simulink model "mapp_4_fir_4_str"  (R2018b)
settings: Solver=ode45  StartTime=0.0  StopTime=200  RelTol=1e-3  EnableMultiTasking=on
undefined symbols (not defined in the file or in its folder): CMD_ci_Re_0, CMD_ci_Re_21, CMD_ci_str_0, CMD_ci_str_1, CMD_ci_str_10, CMD_ci_str_11, CMD_ci_str_12, CMD_ci_str_13, CMD_ci_str_14, CMD_ci_str_15, CMD_ci_str_16, CMD_ci_str_17, CMD_ci_str_18, CMD_ci_str_19, CMD_ci_str_2, CMD_ci_str_20, CMD_ci_str_21, CMD_ci_str_3, CMD_ci_str_4, CMD_ci_str_5, CMD_ci_str_6, CMD_ci_str_7, CMD_ci_str_8, CMD_ci_str_9, CMD_decr_0, CMD_deka_down, CMD_deka_up, CMD_fb, CMD_FB_mult, CMD_Firprg_0, CMD_Firprg_1, CMD_gain, CMD_ind_mult, CMD_ind_mult_1, CMD_ind_mult_2, CMD_ind_mult_3, CMD_ind_mult_4, CMD_ind_stuk, CMD_ind_vol, CMD_ind_vol_1, CMD_ind_vol_2, CMD_ind_vol_3, CMD_ind_vol_4, CMD_init_dac, CMD_init_sw, CMD_molot_string, CMD_nl, CMD_nl_sl, CMD_omega_0, CMD_out_vol, CMD_param_0, CMD_param_5, CMD_pedal, CMD_reset, CMD_rst, CMD_shape_0, CMD_step_down, CMD_step_up, CMD_str_svertk, ind_mult_0 ... (+10)
libraries: xbsIndex_r4 x3300
(part 12 of 16)

== system mapp_4_fir_4_str/Mid_Graph2/Exp/exp-mashinka/gauss0 ==
  sync : Inport
  addr : Inport  Port=2
  Force_vol : Inport  Port=3
  m_data : Inport  Port=4
  m_addr : Inport  Port=5
  m_en : Inport  Port=6
  Addr_ind_vol : Inport  Port=7
  AddSub : xbsIndex_r4/AddSub  mode=Subtraction  use_carryin=off  use_carryout=off  en=off  latency=2  precision=Full  arith_type=Unsigned  n_bits=16  bin_pt=14  quantization=Truncate  overflow=Wrap  use_behavioral_HDL=off  hw_selection=Fabric  pipelined=off  dbl_ovrd=off  block_type=addsub
  Constant1 : xbsIndex_r4/Constant  const=0  gui_display_data_type=Floating-point  arith_type=Floating-point  n_bits=30  bin_pt=0  preci_type=Single  exp_width=8  frac_width=24  explicit_period=on  period=1  equ=P=C  opselect=C  inp2=PCIN>>17  opr=+  inp1=P  carry=CIN  dbl_ovrd=off  block_type=constant
  Constant2 : xbsIndex_r4/Constant  const=30  gui_display_data_type=Floating-point  arith_type=Floating-point  n_bits=16  bin_pt=14  preci_type=Single  exp_width=8  frac_width=24  explicit_period=on  period=1  equ=P=C  opselect=C  inp2=PCIN>>17  opr=+  inp1=P  carry=CIN  dbl_ovrd=off  block_type=constant
  Convert : xbsIndex_r4/Convert  gui_display_data_type=Floating-point  arith_type=Floating-point  n_bits=16  bin_pt=14  float_type=Single  exp_bits=8  fraction_bits=24  quantization=Truncate  overflow=Wrap  en=off  latency=3  pipeline=off  dbl_ovrd=off  block_type=convert
  Convert2 : xbsIndex_r4/Convert  gui_display_data_type=Floating-point  arith_type=Floating-point  n_bits=16  bin_pt=14  float_type=Single  exp_bits=8  fraction_bits=24  quantization=Truncate  overflow=Wrap  en=off  latency=3  pipeline=off  dbl_ovrd=off  block_type=convert
  Convert4 : xbsIndex_r4/Convert  gui_display_data_type=Floating-point  arith_type=Floating-point  n_bits=16  bin_pt=14  float_type=Single  exp_bits=8  fraction_bits=24  quantization=Truncate  overflow=Wrap  en=off  latency=3  pipeline=off  dbl_ovrd=off  block_type=convert
  Delay1 : xbsIndex_r4/Delay  rst=off  infoeditControl=Selection of Reset will increase slice count due to use of real FFs and instead of SRLs  en=off  latency=9  reg_retiming=off  dbl_ovrd=off  block_type=delay
  Delay{2..10,14,18} (11 alike) : xbsIndex_r4/Delay  rst=off  infoeditControl=Selection of Reset will increase slice count due to use of real FFs and instead of SRLs  en=off  latency=1  reg_retiming=off  dbl_ovrd=off  block_type=delay
  Delay11 : xbsIndex_r4/Delay  rst=off  infoeditControl=Selection of Reset will increase slice count due to use of real FFs and instead of SRLs  en=off  latency=14  reg_retiming=off  dbl_ovrd=off  block_type=delay
  Delay12 : xbsIndex_r4/Delay  rst=off  infoeditControl=Selection of Reset will increase slice count due to use of real FFs and instead of SRLs  en=off  latency=2  reg_retiming=off  dbl_ovrd=off  block_type=delay
  Delay13 : xbsIndex_r4/Delay  rst=off  infoeditControl=Selection of Reset will increase slice count due to use of real FFs and instead of SRLs  en=off  latency=8  reg_retiming=off  dbl_ovrd=off  block_type=delay
  Delay15 : xbsIndex_r4/Delay  rst=off  infoeditControl=Selection of Reset will increase slice count due to use of real FFs and instead of SRLs  en=off  latency=9  reg_retiming=off  dbl_ovrd=off  block_type=delay
  Delay16 : xbsIndex_r4/Delay  rst=off  infoeditControl=Selection of Reset will increase slice count due to use of real FFs and instead of SRLs  en=off  latency=8  reg_retiming=off  dbl_ovrd=off  block_type=delay
  Delay17 : xbsIndex_r4/Delay  rst=off  infoeditControl=Selection of Reset will increase slice count due to use of real FFs and instead of SRLs  en=off  latency=3  reg_retiming=off  dbl_ovrd=off  block_type=delay
  Exponential : xbsIndex_r4/Exponential  flow_control=NonBlocking  axi_optimize_goal=Resources  bmg_use=NoUsage  latency=12  has_a_tlast=off  has_a_tuser=off  en=off  has_result_tready=off  has_underflow=on  has_overflow=off  fpo_op_type=exponential  rate=1  has_b_tlast=false  has_b_tuser=false  result_tlast_behv=1  has_divide_by_zero=false  has_invalid_op=false  block_type=exponential
      settings: infoedit=Blocking: Wait for data on all inputs, allow back-pressure.<br>NonBlocking: operate every cycle in which all inputs are valid, no back-pressure.
  Mult : xbsIndex_r4/Mult  precision=Full  arith_type="Signed  (2's comp)"  n_bits=16  bin_pt=14  quantization=Truncate  overflow=Wrap  en=off  latency=6  use_behavioral_HDL=off  opt=Speed  use_embedded=on  optimum_pipeline=off  pipeline=on  dbl_ovrd=off  use_rpm=on  placement_style=Triangular  block_type=mult
  Mult1 : xbsIndex_r4/Mult  precision=Full  arith_type="Signed  (2's comp)"  n_bits=16  bin_pt=14  quantization=Truncate  overflow=Wrap  en=off  latency=6  use_behavioral_HDL=off  opt=Speed  use_embedded=on  optimum_pipeline=off  pipeline=on  dbl_ovrd=off  use_rpm=on  placement_style=Triangular  block_type=mult
  Mult2 : xbsIndex_r4/Mult  precision=Full  arith_type="Signed  (2's comp)"  n_bits=16  bin_pt=14  quantization=Truncate  overflow=Wrap  en=off  latency=6  use_behavioral_HDL=off  opt=Speed  use_embedded=on  optimum_pipeline=off  pipeline=on  dbl_ovrd=off  use_rpm=on  placement_style=Triangular  block_type=mult
  Mux : xbsIndex_r4/Mux  inputs=2  en=off  latency=1  precision=Full  arith_type=Unsigned  n_bits=16  bin_pt=14  quantization=Truncate  overflow=Wrap  dbl_ovrd=off  block_type=mux
  Mux1 : xbsIndex_r4/Mux  inputs=2  en=off  latency=1  precision=Full  arith_type=Unsigned  n_bits=16  bin_pt=14  quantization=Truncate  overflow=Wrap  dbl_ovrd=off  block_type=mux
  Negate : xbsIndex_r4/Negate  precision=Full  arith_type=Unsigned  n_bits=16  bin_pt=14  quantization=Truncate  overflow=Wrap  en=off  latency=1  dbl_ovrd=off  block_type=negate
  Reinterpret : xbsIndex_r4/Reinterpret  force_arith_type=on  arith_type="Signed  (2's comp)"  force_bin_pt=on  bin_pt=29  block_type=reinterpret
  Reinterpret1 : xbsIndex_r4/Reinterpret  force_arith_type=on  arith_type="Signed  (2's comp)"  force_bin_pt=on  bin_pt=18  block_type=reinterpret
  Reinterpret2 : xbsIndex_r4/Reinterpret  force_arith_type=on  arith_type="Signed  (2's comp)"  force_bin_pt=on  bin_pt=24  block_type=reinterpret
  Relational : xbsIndex_r4/Relational  mode=a>=b  op_type=Bool  en=off  latency=3  dbl_ovrd=off  block_type=relational
  exp_a0 : Subsystem
  exp_d0 : Subsystem
  exp_e0 : Subsystem
  z1 : xbsIndex_r4/Delay  rst=off  infoeditControl=Selection of Reset will increase slice count due to use of real FFs and instead of SRLs  en=off  latency=16  reg_retiming=on  dbl_ovrd=off  block_type=delay
      settings: block_version=8.2-EVAL
  z2 : xbsIndex_r4/Delay  rst=off  infoeditControl=Selection of Reset will increase slice count due to use of real FFs and instead of SRLs  en=off  latency=13  reg_retiming=on  dbl_ovrd=off  block_type=delay
      settings: block_version=8.2-EVAL
  z3 : xbsIndex_r4/Delay  rst=off  infoeditControl=Selection of Reset will increase slice count due to use of real FFs and instead of SRLs  en=off  latency=3  reg_retiming=on  dbl_ovrd=off  block_type=delay
      settings: block_version=8.2-EVAL
  Out1 : Outport
  wires:
  z1/1 -> Reinterpret2/1
  z3/1 -> Reinterpret1/1
  exp_d0/1(Out) -> Delay16/1
  Delay15/1 -> Delay2/1
  Delay2/1 -> AddSub/1
  Mux/1 -> Delay8/1
  exp_a0/1(Out) -> z1/1
  Delay7/1 -> Exponential/1
  Delay8/1 -> Mult2/1
  Delay4/1 -> Mult1/2
  Reinterpret2/1 -> Convert2/1
  Convert2/1 -> Delay1/1
  Convert4/1 -> Delay11/1
  Negate/1 -> Delay7/1
  exp_e0/1(Out) -> z3/1
  Reinterpret1/1 -> Convert4/1
  Reinterpret/1 -> Convert/1
  Delay5/1 -> Mult1/1
  Delay10/1 -> Mult2/2
  Constant1/1 -> Mux/2
  AddSub/1 -> Delay3/1
  Delay3/1 -> Reinterpret/1
  Delay11/1 -> Delay4/1
  Delay9/1 -> Out1/1
  addr/1 -> Delay15/1
  Delay12/1 -> Mux/3
  sync/1 -> Mux/1
  Delay14/1 -> Delay13/1
  Delay1/1 -> z2/1
  Delay13/1 -> Delay10/1
  Convert/1 -> Mult/2, Mult/1
  m_data/1 -> exp_d0/2(m_data), exp_a0/2(m_data), exp_e0/2(m_data)
  m_addr/1 -> exp_a0/3(m_addr), exp_d0/3(m_addr), exp_e0/3(m_addr)
  Mult/1 -> Delay5/1
  Exponential/1 -> Delay12/1
  Mult2/1 -> Delay9/1
  Addr_ind_vol/1 -> exp_a0/1(addr), exp_d0/1(addr), exp_e0/1(addr)
  Mult1/1 -> Delay6/1
  m_en/1 -> exp_a0/4(m_en), exp_d0/4(m_en), exp_e0/4(m_en)
  Force_vol/1 -> exp_e0/5(Force_vol), exp_a0/5(Force_vol), exp_d0/5(Force_vol)
  Delay16/1 -> AddSub/2
  z2/1 -> Delay14/1
  Mux1/1 -> Delay18/1
  Constant2/1 -> Relational/2, Mux1/3
  Delay6/1 -> Relational/1, Delay17/1
  Delay17/1 -> Mux1/2
  Relational/1 -> Mux1/1
  Delay18/1 -> Negate/1

== system mapp_4_fir_4_str/Mid_Graph2/Exp/exp-mashinka/gauss1 ==
  sync : Inport
  addr : Inport  Port=2
  Force_vol : Inport  Port=3
  m_data : Inport  Port=4
  m_addr : Inport  Port=5
  m_en : Inport  Port=6
  Addr_ind_vol : Inport  Port=7
  AddSub : xbsIndex_r4/AddSub  mode=Subtraction  use_carryin=off  use_carryout=off  en=off  latency=2  precision=Full  arith_type=Unsigned  n_bits=16  bin_pt=14  quantization=Truncate  overflow=Wrap  use_behavioral_HDL=off  hw_selection=Fabric  pipelined=off  dbl_ovrd=off  block_type=addsub
  Constant1 : xbsIndex_r4/Constant  const=0  gui_display_data_type=Floating-point  arith_type=Floating-point  n_bits=30  bin_pt=0  preci_type=Single  exp_width=8  frac_width=24  explicit_period=on  period=1  equ=P=C  opselect=C  inp2=PCIN>>17  opr=+  inp1=P  carry=CIN  dbl_ovrd=off  block_type=constant
  Constant2 : xbsIndex_r4/Constant  const=30  gui_display_data_type=Floating-point  arith_type=Floating-point  n_bits=16  bin_pt=14  preci_type=Single  exp_width=8  frac_width=24  explicit_period=on  period=1  equ=P=C  opselect=C  inp2=PCIN>>17  opr=+  inp1=P  carry=CIN  dbl_ovrd=off  block_type=constant
  Convert : xbsIndex_r4/Convert  gui_display_data_type=Floating-point  arith_type=Floating-point  n_bits=16  bin_pt=14  float_type=Single  exp_bits=8  fraction_bits=24  quantization=Truncate  overflow=Wrap  en=off  latency=3  pipeline=off  dbl_ovrd=off  block_type=convert
  Convert2 : xbsIndex_r4/Convert  gui_display_data_type=Floating-point  arith_type=Floating-point  n_bits=16  bin_pt=14  float_type=Single  exp_bits=8  fraction_bits=24  quantization=Truncate  overflow=Wrap  en=off  latency=3  pipeline=off  dbl_ovrd=off  block_type=convert
  Convert4 : xbsIndex_r4/Convert  gui_display_data_type=Floating-point  arith_type=Floating-point  n_bits=16  bin_pt=14  float_type=Single  exp_bits=8  fraction_bits=24  quantization=Truncate  overflow=Wrap  en=off  latency=3  pipeline=off  dbl_ovrd=off  block_type=convert
  Delay1 : xbsIndex_r4/Delay  rst=off  infoeditControl=Selection of Reset will increase slice count due to use of real FFs and instead of SRLs  en=off  latency=9  reg_retiming=off  dbl_ovrd=off  block_type=delay
  Delay{2..10,14,18} (11 alike) : xbsIndex_r4/Delay  rst=off  infoeditControl=Selection of Reset will increase slice count due to use of real FFs and instead of SRLs  en=off  latency=1  reg_retiming=off  dbl_ovrd=off  block_type=delay
  Delay11 : xbsIndex_r4/Delay  rst=off  infoeditControl=Selection of Reset will increase slice count due to use of real FFs and instead of SRLs  en=off  latency=14  reg_retiming=off  dbl_ovrd=off  block_type=delay
  Delay12 : xbsIndex_r4/Delay  rst=off  infoeditControl=Selection of Reset will increase slice count due to use of real FFs and instead of SRLs  en=off  latency=2  reg_retiming=off  dbl_ovrd=off  block_type=delay
  Delay13 : xbsIndex_r4/Delay  rst=off  infoeditControl=Selection of Reset will increase slice count due to use of real FFs and instead of SRLs  en=off  latency=8  reg_retiming=off  dbl_ovrd=off  block_type=delay
  Delay15 : xbsIndex_r4/Delay  rst=off  infoeditControl=Selection of Reset will increase slice count due to use of real FFs and instead of SRLs  en=off  latency=9  reg_retiming=off  dbl_ovrd=off  block_type=delay
  Delay16 : xbsIndex_r4/Delay  rst=off  infoeditControl=Selection of Reset will increase slice count due to use of real FFs and instead of SRLs  en=off  latency=8  reg_retiming=off  dbl_ovrd=off  block_type=delay
  Delay17 : xbsIndex_r4/Delay  rst=off  infoeditControl=Selection of Reset will increase slice count due to use of real FFs and instead of SRLs  en=off  latency=3  reg_retiming=off  dbl_ovrd=off  block_type=delay
  Exponential : xbsIndex_r4/Exponential  flow_control=NonBlocking  axi_optimize_goal=Resources  bmg_use=NoUsage  latency=12  has_a_tlast=off  has_a_tuser=off  en=off  has_result_tready=off  has_underflow=on  has_overflow=off  fpo_op_type=exponential  rate=1  has_b_tlast=false  has_b_tuser=false  result_tlast_behv=1  has_divide_by_zero=false  has_invalid_op=false  block_type=exponential
      settings: infoedit=Blocking: Wait for data on all inputs, allow back-pressure.<br>NonBlocking: operate every cycle in which all inputs are valid, no back-pressure.
  Mult : xbsIndex_r4/Mult  precision=Full  arith_type="Signed  (2's comp)"  n_bits=16  bin_pt=14  quantization=Truncate  overflow=Wrap  en=off  latency=6  use_behavioral_HDL=off  opt=Speed  use_embedded=on  optimum_pipeline=off  pipeline=on  dbl_ovrd=off  use_rpm=on  placement_style=Triangular  block_type=mult
  Mult1 : xbsIndex_r4/Mult  precision=Full  arith_type="Signed  (2's comp)"  n_bits=16  bin_pt=14  quantization=Truncate  overflow=Wrap  en=off  latency=6  use_behavioral_HDL=off  opt=Speed  use_embedded=on  optimum_pipeline=off  pipeline=on  dbl_ovrd=off  use_rpm=on  placement_style=Triangular  block_type=mult
  Mult2 : xbsIndex_r4/Mult  precision=Full  arith_type="Signed  (2's comp)"  n_bits=16  bin_pt=14  quantization=Truncate  overflow=Wrap  en=off  latency=6  use_behavioral_HDL=off  opt=Speed  use_embedded=on  optimum_pipeline=off  pipeline=on  dbl_ovrd=off  use_rpm=on  placement_style=Triangular  block_type=mult
  Mux : xbsIndex_r4/Mux  inputs=2  en=off  latency=1  precision=Full  arith_type=Unsigned  n_bits=16  bin_pt=14  quantization=Truncate  overflow=Wrap  dbl_ovrd=off  block_type=mux
  Mux1 : xbsIndex_r4/Mux  inputs=2  en=off  latency=1  precision=Full  arith_type=Unsigned  n_bits=16  bin_pt=14  quantization=Truncate  overflow=Wrap  dbl_ovrd=off  block_type=mux
  Negate : xbsIndex_r4/Negate  precision=Full  arith_type=Unsigned  n_bits=16  bin_pt=14  quantization=Truncate  overflow=Wrap  en=off  latency=1  dbl_ovrd=off  block_type=negate
  Reinterpret : xbsIndex_r4/Reinterpret  force_arith_type=on  arith_type="Signed  (2's comp)"  force_bin_pt=on  bin_pt=29  block_type=reinterpret
  Reinterpret1 : xbsIndex_r4/Reinterpret  force_arith_type=on  arith_type="Signed  (2's comp)"  force_bin_pt=on  bin_pt=18  block_type=reinterpret
  Reinterpret2 : xbsIndex_r4/Reinterpret  force_arith_type=on  arith_type="Signed  (2's comp)"  force_bin_pt=on  bin_pt=24  block_type=reinterpret
  Relational : xbsIndex_r4/Relational  mode=a>=b  op_type=Bool  en=off  latency=3  dbl_ovrd=off  block_type=relational
  exp_a0 : Subsystem
  exp_d0 : Subsystem
  exp_e0 : Subsystem
  z1 : xbsIndex_r4/Delay  rst=off  infoeditControl=Selection of Reset will increase slice count due to use of real FFs and instead of SRLs  en=off  latency=16  reg_retiming=on  dbl_ovrd=off  block_type=delay
      settings: block_version=8.2-EVAL
  z2 : xbsIndex_r4/Delay  rst=off  infoeditControl=Selection of Reset will increase slice count due to use of real FFs and instead of SRLs  en=off  latency=13  reg_retiming=on  dbl_ovrd=off  block_type=delay
      settings: block_version=8.2-EVAL
  z3 : xbsIndex_r4/Delay  rst=off  infoeditControl=Selection of Reset will increase slice count due to use of real FFs and instead of SRLs  en=off  latency=3  reg_retiming=on  dbl_ovrd=off  block_type=delay
      settings: block_version=8.2-EVAL
  Out1 : Outport
  wires:
  z2/1 -> Delay14/1
  Delay16/1 -> AddSub/2
  Force_vol/1 -> exp_d0/5(Force_vol), exp_a0/5(Force_vol), exp_e0/5(Force_vol)
  m_en/1 -> exp_e0/4(m_en), exp_d0/4(m_en), exp_a0/4(m_en)
  Mult1/1 -> Delay6/1
  Addr_ind_vol/1 -> exp_e0/1(addr), exp_d0/1(addr), exp_a0/1(addr)
  Mult2/1 -> Delay9/1
  Exponential/1 -> Delay12/1
  Mult/1 -> Delay5/1
  m_addr/1 -> exp_e0/3(m_addr), exp_d0/3(m_addr), exp_a0/3(m_addr)
  m_data/1 -> exp_e0/2(m_data), exp_a0/2(m_data), exp_d0/2(m_data)
  Convert/1 -> Mult/1, Mult/2
  Delay13/1 -> Delay10/1
  Delay1/1 -> z2/1
  Delay14/1 -> Delay13/1
  sync/1 -> Mux/1
  Delay12/1 -> Mux/3
  addr/1 -> Delay15/1
  Delay9/1 -> Out1/1
  Delay11/1 -> Delay4/1
  Delay3/1 -> Reinterpret/1
  AddSub/1 -> Delay3/1
  Constant1/1 -> Mux/2
  Delay10/1 -> Mult2/2
  Delay5/1 -> Mult1/1
  Reinterpret/1 -> Convert/1
  Reinterpret1/1 -> Convert4/1
  exp_e0/1(Out) -> z3/1
  Negate/1 -> Delay7/1
  Convert4/1 -> Delay11/1
  Convert2/1 -> Delay1/1
  Reinterpret2/1 -> Convert2/1
  Delay4/1 -> Mult1/2
  Delay8/1 -> Mult2/1
  Delay7/1 -> Exponential/1
  exp_a0/1(Out) -> z1/1
  Mux/1 -> Delay8/1
  Delay2/1 -> AddSub/1
  Delay15/1 -> Delay2/1
  exp_d0/1(Out) -> Delay16/1
  z3/1 -> Reinterpret1/1
  z1/1 -> Reinterpret2/1
  Delay6/1 -> Relational/1, Delay17/1
  Constant2/1 -> Relational/2, Mux1/3
  Relational/1 -> Mux1/1
  Delay17/1 -> Mux1/2
  Mux1/1 -> Delay18/1
  Delay18/1 -> Negate/1

== system mapp_4_fir_4_str/Mid_Graph2/Exp/exp-mashinka/gauss2 ==
  sync : Inport
  addr : Inport  Port=2
  Force_vol : Inport  Port=3
  m_data : Inport  Port=4
  m_addr : Inport  Port=5
  m_en : Inport  Port=6
  Addr_ind_vol : Inport  Port=7
  AddSub : xbsIndex_r4/AddSub  mode=Subtraction  use_carryin=off  use_carryout=off  en=off  latency=2  precision=Full  arith_type=Unsigned  n_bits=16  bin_pt=14  quantization=Truncate  overflow=Wrap  use_behavioral_HDL=off  hw_selection=Fabric  pipelined=off  dbl_ovrd=off  block_type=addsub
  Constant1 : xbsIndex_r4/Constant  const=0  gui_display_data_type=Floating-point  arith_type=Floating-point  n_bits=30  bin_pt=0  preci_type=Single  exp_width=8  frac_width=24  explicit_period=on  period=1  equ=P=C  opselect=C  inp2=PCIN>>17  opr=+  inp1=P  carry=CIN  dbl_ovrd=off  block_type=constant
  Constant2 : xbsIndex_r4/Constant  const=30  gui_display_data_type=Floating-point  arith_type=Floating-point  n_bits=16  bin_pt=14  preci_type=Single  exp_width=8  frac_width=24  explicit_period=on  period=1  equ=P=C  opselect=C  inp2=PCIN>>17  opr=+  inp1=P  carry=CIN  dbl_ovrd=off  block_type=constant
  Convert : xbsIndex_r4/Convert  gui_display_data_type=Floating-point  arith_type=Floating-point  n_bits=16  bin_pt=14  float_type=Single  exp_bits=8  fraction_bits=24  quantization=Truncate  overflow=Wrap  en=off  latency=3  pipeline=off  dbl_ovrd=off  block_type=convert
  Convert2 : xbsIndex_r4/Convert  gui_display_data_type=Floating-point  arith_type=Floating-point  n_bits=16  bin_pt=14  float_type=Single  exp_bits=8  fraction_bits=24  quantization=Truncate  overflow=Wrap  en=off  latency=3  pipeline=off  dbl_ovrd=off  block_type=convert
  Convert4 : xbsIndex_r4/Convert  gui_display_data_type=Floating-point  arith_type=Floating-point  n_bits=16  bin_pt=14  float_type=Single  exp_bits=8  fraction_bits=24  quantization=Truncate  overflow=Wrap  en=off  latency=3  pipeline=off  dbl_ovrd=off  block_type=convert
  Delay1 : xbsIndex_r4/Delay  rst=off  infoeditControl=Selection of Reset will increase slice count due to use of real FFs and instead of SRLs  en=off  latency=9  reg_retiming=off  dbl_ovrd=off  block_type=delay
  Delay{2..10,14,18} (11 alike) : xbsIndex_r4/Delay  rst=off  infoeditControl=Selection of Reset will increase slice count due to use of real FFs and instead of SRLs  en=off  latency=1  reg_retiming=off  dbl_ovrd=off  block_type=delay
  Delay11 : xbsIndex_r4/Delay  rst=off  infoeditControl=Selection of Reset will increase slice count due to use of real FFs and instead of SRLs  en=off  latency=14  reg_retiming=off  dbl_ovrd=off  block_type=delay
  Delay12 : xbsIndex_r4/Delay  rst=off  infoeditControl=Selection of Reset will increase slice count due to use of real FFs and instead of SRLs  en=off  latency=2  reg_retiming=off  dbl_ovrd=off  block_type=delay
  Delay13 : xbsIndex_r4/Delay  rst=off  infoeditControl=Selection of Reset will increase slice count due to use of real FFs and instead of SRLs  en=off  latency=8  reg_retiming=off  dbl_ovrd=off  block_type=delay
  Delay15 : xbsIndex_r4/Delay  rst=off  infoeditControl=Selection of Reset will increase slice count due to use of real FFs and instead of SRLs  en=off  latency=9  reg_retiming=off  dbl_ovrd=off  block_type=delay
  Delay16 : xbsIndex_r4/Delay  rst=off  infoeditControl=Selection of Reset will increase slice count due to use of real FFs and instead of SRLs  en=off  latency=8  reg_retiming=off  dbl_ovrd=off  block_type=delay
  Delay17 : xbsIndex_r4/Delay  rst=off  infoeditControl=Selection of Reset will increase slice count due to use of real FFs and instead of SRLs  en=off  latency=3  reg_retiming=off  dbl_ovrd=off  block_type=delay
  Exponential : xbsIndex_r4/Exponential  flow_control=NonBlocking  axi_optimize_goal=Resources  bmg_use=NoUsage  latency=12  has_a_tlast=off  has_a_tuser=off  en=off  has_result_tready=off  has_underflow=on  has_overflow=off  fpo_op_type=exponential  rate=1  has_b_tlast=false  has_b_tuser=false  result_tlast_behv=1  has_divide_by_zero=false  has_invalid_op=false  block_type=exponential
      settings: infoedit=Blocking: Wait for data on all inputs, allow back-pressure.<br>NonBlocking: operate every cycle in which all inputs are valid, no back-pressure.
  Mult : xbsIndex_r4/Mult  precision=Full  arith_type="Signed  (2's comp)"  n_bits=16  bin_pt=14  quantization=Truncate  overflow=Wrap  en=off  latency=6  use_behavioral_HDL=off  opt=Speed  use_embedded=on  optimum_pipeline=off  pipeline=on  dbl_ovrd=off  use_rpm=on  placement_style=Triangular  block_type=mult
  Mult1 : xbsIndex_r4/Mult  precision=Full  arith_type="Signed  (2's comp)"  n_bits=16  bin_pt=14  quantization=Truncate  overflow=Wrap  en=off  latency=6  use_behavioral_HDL=off  opt=Speed  use_embedded=on  optimum_pipeline=off  pipeline=on  dbl_ovrd=off  use_rpm=on  placement_style=Triangular  block_type=mult
  Mult2 : xbsIndex_r4/Mult  precision=Full  arith_type="Signed  (2's comp)"  n_bits=16  bin_pt=14  quantization=Truncate  overflow=Wrap  en=off  latency=6  use_behavioral_HDL=off  opt=Speed  use_embedded=on  optimum_pipeline=off  pipeline=on  dbl_ovrd=off  use_rpm=on  placement_style=Triangular  block_type=mult
  Mux : xbsIndex_r4/Mux  inputs=2  en=off  latency=1  precision=Full  arith_type=Unsigned  n_bits=16  bin_pt=14  quantization=Truncate  overflow=Wrap  dbl_ovrd=off  block_type=mux
  Mux1 : xbsIndex_r4/Mux  inputs=2  en=off  latency=1  precision=Full  arith_type=Unsigned  n_bits=16  bin_pt=14  quantization=Truncate  overflow=Wrap  dbl_ovrd=off  block_type=mux
  Negate : xbsIndex_r4/Negate  precision=Full  arith_type=Unsigned  n_bits=16  bin_pt=14  quantization=Truncate  overflow=Wrap  en=off  latency=1  dbl_ovrd=off  block_type=negate
  Reinterpret : xbsIndex_r4/Reinterpret  force_arith_type=on  arith_type="Signed  (2's comp)"  force_bin_pt=on  bin_pt=29  block_type=reinterpret
  Reinterpret1 : xbsIndex_r4/Reinterpret  force_arith_type=on  arith_type="Signed  (2's comp)"  force_bin_pt=on  bin_pt=18  block_type=reinterpret
  Reinterpret2 : xbsIndex_r4/Reinterpret  force_arith_type=on  arith_type="Signed  (2's comp)"  force_bin_pt=on  bin_pt=24  block_type=reinterpret
  Relational : xbsIndex_r4/Relational  mode=a>=b  op_type=Bool  en=off  latency=3  dbl_ovrd=off  block_type=relational
  exp_a0 : Subsystem
  exp_d0 : Subsystem
  exp_e0 : Subsystem
  z1 : xbsIndex_r4/Delay  rst=off  infoeditControl=Selection of Reset will increase slice count due to use of real FFs and instead of SRLs  en=off  latency=16  reg_retiming=on  dbl_ovrd=off  block_type=delay
      settings: block_version=8.2-EVAL
  z2 : xbsIndex_r4/Delay  rst=off  infoeditControl=Selection of Reset will increase slice count due to use of real FFs and instead of SRLs  en=off  latency=13  reg_retiming=on  dbl_ovrd=off  block_type=delay
      settings: block_version=8.2-EVAL
  z3 : xbsIndex_r4/Delay  rst=off  infoeditControl=Selection of Reset will increase slice count due to use of real FFs and instead of SRLs  en=off  latency=3  reg_retiming=on  dbl_ovrd=off  block_type=delay
      settings: block_version=8.2-EVAL
  Out1 : Outport
  wires:
  z1/1 -> Reinterpret2/1
  z3/1 -> Reinterpret1/1
  exp_d0/1(Out) -> Delay16/1
  Delay15/1 -> Delay2/1
  Delay2/1 -> AddSub/1
  Mux/1 -> Delay8/1
  exp_a0/1(Out) -> z1/1
  Delay7/1 -> Exponential/1
  Delay8/1 -> Mult2/1
  Delay4/1 -> Mult1/2
  Reinterpret2/1 -> Convert2/1
  Convert2/1 -> Delay1/1
  Convert4/1 -> Delay11/1
  Negate/1 -> Delay7/1
  exp_e0/1(Out) -> z3/1
  Reinterpret1/1 -> Convert4/1
  Reinterpret/1 -> Convert/1
  Delay5/1 -> Mult1/1
  Delay10/1 -> Mult2/2
  Constant1/1 -> Mux/2
  AddSub/1 -> Delay3/1
  Delay3/1 -> Reinterpret/1
  Delay11/1 -> Delay4/1
  Delay9/1 -> Out1/1
  addr/1 -> Delay15/1
  Delay12/1 -> Mux/3
  sync/1 -> Mux/1
  Delay14/1 -> Delay13/1
  Delay1/1 -> z2/1
  Delay13/1 -> Delay10/1
  Convert/1 -> Mult/2, Mult/1
  m_data/1 -> exp_d0/2(m_data), exp_a0/2(m_data), exp_e0/2(m_data)
  m_addr/1 -> exp_a0/3(m_addr), exp_d0/3(m_addr), exp_e0/3(m_addr)
  Mult/1 -> Delay5/1
  Exponential/1 -> Delay12/1
  Mult2/1 -> Delay9/1
  Addr_ind_vol/1 -> exp_a0/1(addr), exp_d0/1(addr), exp_e0/1(addr)
  Mult1/1 -> Delay6/1
  m_en/1 -> exp_a0/4(m_en), exp_d0/4(m_en), exp_e0/4(m_en)
  Force_vol/1 -> exp_e0/5(Force_vol), exp_a0/5(Force_vol), exp_d0/5(Force_vol)
  Delay16/1 -> AddSub/2
  z2/1 -> Delay14/1
  Delay6/1 -> Relational/1, Delay17/1
  Delay17/1 -> Mux1/2
  Relational/1 -> Mux1/1
  Mux1/1 -> Delay18/1
  Constant2/1 -> Relational/2, Mux1/3
  Delay18/1 -> Negate/1

== system mapp_4_fir_4_str/Mid_Graph2/Exp/exp-mashinka/gauss3 ==
  sync : Inport
  addr : Inport  Port=2
  Force_vol : Inport  Port=3
  m_data : Inport  Port=4
  m_addr : Inport  Port=5
  m_en : Inport  Port=6
  Addr_ind_vol : Inport  Port=7
  AddSub : xbsIndex_r4/AddSub  mode=Subtraction  use_carryin=off  use_carryout=off  en=off  latency=2  precision=Full  arith_type=Unsigned  n_bits=16  bin_pt=14  quantization=Truncate  overflow=Wrap  use_behavioral_HDL=off  hw_selection=Fabric  pipelined=off  dbl_ovrd=off  block_type=addsub
  Constant1 : xbsIndex_r4/Constant  const=0  gui_display_data_type=Floating-point  arith_type=Floating-point  n_bits=30  bin_pt=0  preci_type=Single  exp_width=8  frac_width=24  explicit_period=on  period=1  equ=P=C  opselect=C  inp2=PCIN>>17  opr=+  inp1=P  carry=CIN  dbl_ovrd=off  block_type=constant
  Constant2 : xbsIndex_r4/Constant  const=30  gui_display_data_type=Floating-point  arith_type=Floating-point  n_bits=16  bin_pt=14  preci_type=Single  exp_width=8  frac_width=24  explicit_period=on  period=1  equ=P=C  opselect=C  inp2=PCIN>>17  opr=+  inp1=P  carry=CIN  dbl_ovrd=off  block_type=constant
  Convert : xbsIndex_r4/Convert  gui_display_data_type=Floating-point  arith_type=Floating-point  n_bits=16  bin_pt=14  float_type=Single  exp_bits=8  fraction_bits=24  quantization=Truncate  overflow=Wrap  en=off  latency=3  pipeline=off  dbl_ovrd=off  block_type=convert
  Convert2 : xbsIndex_r4/Convert  gui_display_data_type=Floating-point  arith_type=Floating-point  n_bits=16  bin_pt=14  float_type=Single  exp_bits=8  fraction_bits=24  quantization=Truncate  overflow=Wrap  en=off  latency=3  pipeline=off  dbl_ovrd=off  block_type=convert
  Convert4 : xbsIndex_r4/Convert  gui_display_data_type=Floating-point  arith_type=Floating-point  n_bits=16  bin_pt=14  float_type=Single  exp_bits=8  fraction_bits=24  quantization=Truncate  overflow=Wrap  en=off  latency=3  pipeline=off  dbl_ovrd=off  block_type=convert
  Delay1 : xbsIndex_r4/Delay  rst=off  infoeditControl=Selection of Reset will increase slice count due to use of real FFs and instead of SRLs  en=off  latency=9  reg_retiming=off  dbl_ovrd=off  block_type=delay
  Delay{2..10,14,18} (11 alike) : xbsIndex_r4/Delay  rst=off  infoeditControl=Selection of Reset will increase slice count due to use of real FFs and instead of SRLs  en=off  latency=1  reg_retiming=off  dbl_ovrd=off  block_type=delay
  Delay11 : xbsIndex_r4/Delay  rst=off  infoeditControl=Selection of Reset will increase slice count due to use of real FFs and instead of SRLs  en=off  latency=14  reg_retiming=off  dbl_ovrd=off  block_type=delay
  Delay12 : xbsIndex_r4/Delay  rst=off  infoeditControl=Selection of Reset will increase slice count due to use of real FFs and instead of SRLs  en=off  latency=2  reg_retiming=off  dbl_ovrd=off  block_type=delay
  Delay13 : xbsIndex_r4/Delay  rst=off  infoeditControl=Selection of Reset will increase slice count due to use of real FFs and instead of SRLs  en=off  latency=8  reg_retiming=off  dbl_ovrd=off  block_type=delay
  Delay15 : xbsIndex_r4/Delay  rst=off  infoeditControl=Selection of Reset will increase slice count due to use of real FFs and instead of SRLs  en=off  latency=9  reg_retiming=off  dbl_ovrd=off  block_type=delay
  Delay16 : xbsIndex_r4/Delay  rst=off  infoeditControl=Selection of Reset will increase slice count due to use of real FFs and instead of SRLs  en=off  latency=8  reg_retiming=off  dbl_ovrd=off  block_type=delay
  Delay17 : xbsIndex_r4/Delay  rst=off  infoeditControl=Selection of Reset will increase slice count due to use of real FFs and instead of SRLs  en=off  latency=3  reg_retiming=off  dbl_ovrd=off  block_type=delay
  Exponential : xbsIndex_r4/Exponential  flow_control=NonBlocking  axi_optimize_goal=Resources  bmg_use=NoUsage  latency=12  has_a_tlast=off  has_a_tuser=off  en=off  has_result_tready=off  has_underflow=on  has_overflow=off  fpo_op_type=exponential  rate=1  has_b_tlast=false  has_b_tuser=false  result_tlast_behv=1  has_divide_by_zero=false  has_invalid_op=false  block_type=exponential
      settings: infoedit=Blocking: Wait for data on all inputs, allow back-pressure.<br>NonBlocking: operate every cycle in which all inputs are valid, no back-pressure.
  Mult : xbsIndex_r4/Mult  precision=Full  arith_type="Signed  (2's comp)"  n_bits=16  bin_pt=14  quantization=Truncate  overflow=Wrap  en=off  latency=6  use_behavioral_HDL=off  opt=Speed  use_embedded=on  optimum_pipeline=off  pipeline=on  dbl_ovrd=off  use_rpm=on  placement_style=Triangular  block_type=mult
  Mult1 : xbsIndex_r4/Mult  precision=Full  arith_type="Signed  (2's comp)"  n_bits=16  bin_pt=14  quantization=Truncate  overflow=Wrap  en=off  latency=6  use_behavioral_HDL=off  opt=Speed  use_embedded=on  optimum_pipeline=off  pipeline=on  dbl_ovrd=off  use_rpm=on  placement_style=Triangular  block_type=mult
  Mult2 : xbsIndex_r4/Mult  precision=Full  arith_type="Signed  (2's comp)"  n_bits=16  bin_pt=14  quantization=Truncate  overflow=Wrap  en=off  latency=6  use_behavioral_HDL=off  opt=Speed  use_embedded=on  optimum_pipeline=off  pipeline=on  dbl_ovrd=off  use_rpm=on  placement_style=Triangular  block_type=mult
  Mux : xbsIndex_r4/Mux  inputs=2  en=off  latency=1  precision=Full  arith_type=Unsigned  n_bits=16  bin_pt=14  quantization=Truncate  overflow=Wrap  dbl_ovrd=off  block_type=mux
  Mux1 : xbsIndex_r4/Mux  inputs=2  en=off  latency=1  precision=Full  arith_type=Unsigned  n_bits=16  bin_pt=14  quantization=Truncate  overflow=Wrap  dbl_ovrd=off  block_type=mux
  Negate : xbsIndex_r4/Negate  precision=Full  arith_type=Unsigned  n_bits=16  bin_pt=14  quantization=Truncate  overflow=Wrap  en=off  latency=1  dbl_ovrd=off  block_type=negate
  Reinterpret : xbsIndex_r4/Reinterpret  force_arith_type=on  arith_type="Signed  (2's comp)"  force_bin_pt=on  bin_pt=29  block_type=reinterpret
  Reinterpret1 : xbsIndex_r4/Reinterpret  force_arith_type=on  arith_type="Signed  (2's comp)"  force_bin_pt=on  bin_pt=18  block_type=reinterpret
  Reinterpret2 : xbsIndex_r4/Reinterpret  force_arith_type=on  arith_type="Signed  (2's comp)"  force_bin_pt=on  bin_pt=24  block_type=reinterpret
  Relational : xbsIndex_r4/Relational  mode=a>=b  op_type=Bool  en=off  latency=3  dbl_ovrd=off  block_type=relational
  exp_a0 : Subsystem
  exp_d0 : Subsystem
  exp_e0 : Subsystem
  z1 : xbsIndex_r4/Delay  rst=off  infoeditControl=Selection of Reset will increase slice count due to use of real FFs and instead of SRLs  en=off  latency=16  reg_retiming=on  dbl_ovrd=off  block_type=delay
      settings: block_version=8.2-EVAL
  z2 : xbsIndex_r4/Delay  rst=off  infoeditControl=Selection of Reset will increase slice count due to use of real FFs and instead of SRLs  en=off  latency=13  reg_retiming=on  dbl_ovrd=off  block_type=delay
      settings: block_version=8.2-EVAL
  z3 : xbsIndex_r4/Delay  rst=off  infoeditControl=Selection of Reset will increase slice count due to use of real FFs and instead of SRLs  en=off  latency=3  reg_retiming=on  dbl_ovrd=off  block_type=delay
      settings: block_version=8.2-EVAL
  Out1 : Outport
  wires:
  z2/1 -> Delay14/1
  Delay16/1 -> AddSub/2
  Force_vol/1 -> exp_d0/5(Force_vol), exp_a0/5(Force_vol), exp_e0/5(Force_vol)
  m_en/1 -> exp_e0/4(m_en), exp_d0/4(m_en), exp_a0/4(m_en)
  Mult1/1 -> Delay6/1
  Addr_ind_vol/1 -> exp_e0/1(addr), exp_d0/1(addr), exp_a0/1(addr)
  Mult2/1 -> Delay9/1
  Exponential/1 -> Delay12/1
  Mult/1 -> Delay5/1
  m_addr/1 -> exp_e0/3(m_addr), exp_d0/3(m_addr), exp_a0/3(m_addr)
  m_data/1 -> exp_e0/2(m_data), exp_a0/2(m_data), exp_d0/2(m_data)
  Convert/1 -> Mult/1, Mult/2
  Delay13/1 -> Delay10/1
  Delay1/1 -> z2/1
  Delay14/1 -> Delay13/1
  sync/1 -> Mux/1
  Delay12/1 -> Mux/3
  addr/1 -> Delay15/1
  Delay9/1 -> Out1/1
  Delay11/1 -> Delay4/1
  Delay3/1 -> Reinterpret/1
  AddSub/1 -> Delay3/1
  Constant1/1 -> Mux/2
  Delay10/1 -> Mult2/2
  Delay5/1 -> Mult1/1
  Reinterpret/1 -> Convert/1
  Reinterpret1/1 -> Convert4/1
  exp_e0/1(Out) -> z3/1
  Negate/1 -> Delay7/1
  Convert4/1 -> Delay11/1
  Convert2/1 -> Delay1/1
  Reinterpret2/1 -> Convert2/1
  Delay4/1 -> Mult1/2
  Delay8/1 -> Mult2/1
  Delay7/1 -> Exponential/1
  exp_a0/1(Out) -> z1/1
  Mux/1 -> Delay8/1
  Delay2/1 -> AddSub/1
  Delay15/1 -> Delay2/1
  exp_d0/1(Out) -> Delay16/1
  z3/1 -> Reinterpret1/1
  z1/1 -> Reinterpret2/1
  Delay6/1 -> Relational/1, Delay17/1
  Delay17/1 -> Mux1/2
  Relational/1 -> Mux1/1
  Mux1/1 -> Delay18/1
  Constant2/1 -> Relational/2, Mux1/3
  Delay18/1 -> Negate/1

== system mapp_4_fir_4_str/mashinka_0/Force_str0/PARAMETERS/Subsystem1 ==
  addr : Inport
  str_we : Inport  Port=2
  addr_prg : Inport  Port=3
  Imax4 : xbsIndex_r4/Delay  rst=off  infoeditControl=Selection of Reset will increase slice count due to use of real FFs and instead of SRLs  en=off  latency=1  reg_retiming=off  dbl_ovrd=off  block_type=delay
      settings: infoedit=Hardware notes: A delay line is a chain, each link of which is an SRL16 followed by a flip-flop. If register retiming is enabled, the delay line is a chain of flip-flops.  xl_area=[1 1 0 1 0 0 0]  block_version=VER_STRING_GOES_HERE
  Logical : xbsIndex_r4/Logical  logical_function=OR  inputs=2  en=off  latency=0  precision=Full  arith_type=Unsigned  n_bits=16  bin_pt=0  align_bp=on  dbl_ovrd=off  block_type=logical
  Register1 : xbsIndex_r4/Register  init=0  rst=on  en=on  dbl_ovrd=off  block_type=register
      settings: block_version=8.2-EVAL
  Register4 : xbsIndex_r4/Register  init=0  rst=on  en=on  dbl_ovrd=off  block_type=register
      settings: block_version=8.2-EVAL
  Register5 : xbsIndex_r4/Register  init=0  rst=off  en=off  dbl_ovrd=off  block_type=register
  Relational14 : xbsIndex_r4/Relational  mode=a=b  op_type=Bool  en=off  latency=0  dbl_ovrd=off  block_type=relational
  Relational2 : xbsIndex_r4/Relational  mode=a=b  op_type=Bool  en=off  latency=0  dbl_ovrd=off  block_type=relational
  Subsystem : Subsystem
  Subsystem1 : Subsystem
  c3 : xbsIndex_r4/Constant  const=1  gui_display_data_type=Boolean  arith_type=Boolean  n_bits=8  bin_pt=0  preci_type=Single  exp_width=8  frac_width=24  explicit_period=on  period=1  equ=P=C  opselect=C  inp2=PCIN>>17  opr=+  inp1=P  carry=CIN  dbl_ovrd=off  block_type=constant
      settings: block_version=VER_STRING_GOES_HERE
  en1 : Subsystem
  prm0 : xbsIndex_r4/Constant  const=prm0  gui_display_data_type=Fixed-point  arith_type=Unsigned  n_bits=8  bin_pt=0  preci_type=Single  exp_width=8  frac_width=24  explicit_period=on  period=1  equ=P=C  opselect=C  inp2=PCIN>>17  opr=+  inp1=P  carry=CIN  dbl_ovrd=off  block_type=constant
      settings: block_version=VER_STRING_GOES_HERE
  prm1 : xbsIndex_r4/Constant  const=prm0  gui_display_data_type=Fixed-point  arith_type=Unsigned  n_bits=8  bin_pt=0  preci_type=Single  exp_width=8  frac_width=24  explicit_period=on  period=1  equ=P=C  opselect=C  inp2=PCIN>>17  opr=+  inp1=P  carry=CIN  dbl_ovrd=off  block_type=constant
      settings: block_version=VER_STRING_GOES_HERE
  Out2 : Outport
  wires:
  c3/1 -> Register1/1
  prm1/1 -> Relational14/2
  Register5/1 -> Register4/2
  en1/1(Out1) -> Register4/3, Register5/1
  addr/1 -> Relational2/1
  addr_prg/1 -> Relational2/2
  Relational2/1 -> Subsystem/1(In1)
  Subsystem/2(fall) -> Register1/2
  Register1/1 -> Subsystem1/1(In1)
  str_we/1 -> en1/1(In1)
  prm0/1 -> Register4/1
  Register4/1 -> Relational14/1
  Subsystem1/1(rise) -> ?
  Subsystem1/2(fall) -> Out2/1
  Imax4/1 -> Logical/2
  Relational14/1 -> Logical/1, Imax4/1
  Logical/1 -> Register1/3

== system mapp_4_fir_4_str/mashinka_0/Force_str0/PARAMETERS/Subsystem2 ==
  In1 : Inport
  Constant1 : xbsIndex_r4/Constant  const=num_point_256 - 32 + 10  gui_display_data_type=Fixed-point  arith_type=Unsigned  n_bits=ceil(log2(num_point_256))  bin_pt=0  preci_type=Single  exp_width=8  frac_width=24  explicit_period=on  period=1  equ=P=C  opselect=C  inp2=PCIN>>17  opr=+  inp1=P  carry=CIN  dbl_ovrd=off  block_type=constant
      settings: block_version=VER_STRING_GOES_HERE
  Counter6 : xbsIndex_r4/Counter  cnt_type=Count Limited  cnt_to=11  operation=Up  start_count=0  cnt_by_val=1  arith_type=Unsigned  n_bits=4  bin_pt=0  load_pin=off  rst=off  en=on  explicit_period=on  period=1  use_behavioral_HDL=off  implementation=Fabric  use_rpm=off  dbl_ovrd=off  block_type=counter
      settings: block_version=8.2.02
  Logical : xbsIndex_r4/Logical  logical_function=OR  inputs=12  en=off  latency=0  precision=Full  arith_type=Unsigned  n_bits=16  bin_pt=0  align_bp=on  dbl_ovrd=off  block_type=logical
  RSlice6 : xbsIndex_r4/Slice  nbits=ceil(log2(num_point_256 - 1));  boolean_output=off  mode=Lower Bit Location + Width  bit1=0  base1=MSB of Input  bit0=0  base0=LSB of Input  dbl_ovrd=off  block_type=slice
      settings: block_version=VER_STRING_GOES_HERE
  Relational5 : xbsIndex_r4/Relational  mode=a=b  op_type=Bool  en=off  latency=2  dbl_ovrd=off  block_type=relational
      settings: xl_area=[3 1 0 6 0 0 0]  block_version=VER_STRING_GOES_HERE
  Scope1 : Scope  NumInputPorts=9
  prg{1..11} (11 alike) : xbsIndex_r4/Delay  rst=off  infoeditControl=Selection of Reset will increase slice count due to use of real FFs and instead of SRLs  en=off  latency=1  reg_retiming=on  dbl_ovrd=off  block_type=delay
      settings: infoedit=Hardware notes: A delay line is a chain, each link of which is an SRL16 followed by a flip-flop. If register retiming is enabled, the delay line is a chain of flip-flops.  block_version=8.2-EVAL
  strb : Outport
  Out1 : Outport  Port=2
  wires:
  Counter6/1 -> Scope1/5, Out1/1
  prg2/1 -> Logical/8, prg3/1
  prg1/1 -> prg2/1, Logical/7
  In1/1 -> Scope1/1, RSlice6/1
  Logical/1 -> Scope1/4, Counter6/1
  prg8/1 -> prg1/1, Logical/6
  prg7/1 -> prg8/1, Logical/5
  prg6/1 -> prg7/1, Logical/4
  prg5/1 -> prg6/1, Logical/3
  prg4/1 -> prg5/1, Logical/2
  Relational5/1 -> Scope1/3, strb/1, Logical/1, prg4/1
  Constant1/1 -> Relational5/2
  RSlice6/1 -> Scope1/2, Relational5/1
  prg3/1 -> prg9/1, Logical/9
  prg9/1 -> prg10/1, Logical/10
  prg10/1 -> prg11/1, Logical/11
  prg11/1 -> Logical/12

== system mapp_4_fir_4_str/mashinka_0/Force_str0/PARAMETERS/Subsystem3 ==
  count_in : Inport
  Counter1 : xbsIndex_r4/Counter  cnt_type=Count Limited  cnt_to=11  operation=Up  start_count=0  cnt_by_val=1  arith_type=Unsigned  n_bits=4  bin_pt=0  load_pin=off  rst=off  en=on  explicit_period=on  period=1  use_behavioral_HDL=off  implementation=Fabric  use_rpm=off  dbl_ovrd=off  block_type=counter
      settings: block_version=8.2.02
  Counter2 : xbsIndex_r4/Counter  cnt_type=Count Limited  cnt_to=3  operation=Up  start_count=0  cnt_by_val=1  arith_type=Unsigned  n_bits=2  bin_pt=0  load_pin=off  rst=off  en=on  explicit_period=on  period=1  use_behavioral_HDL=off  implementation=Fabric  use_rpm=off  dbl_ovrd=off  block_type=counter
      settings: block_version=8.2.02
  Logical1 : xbsIndex_r4/Logical  logical_function=OR  inputs=4  en=off  latency=1  precision=Full  arith_type=Unsigned  n_bits=16  bin_pt=0  align_bp=on  dbl_ovrd=off  block_type=logical
  Logical2 : xbsIndex_r4/Logical  logical_function=OR  inputs=12  en=off  latency=0  precision=Full  arith_type=Unsigned  n_bits=16  bin_pt=0  align_bp=on  dbl_ovrd=off  block_type=logical
  Relational{1..4} (4 alike) : xbsIndex_r4/Relational  mode=a=b  op_type=Bool  en=off  latency=1  dbl_ovrd=off  block_type=relational
      settings: xl_area=[3 1 0 6 0 0 0]  block_version=VER_STRING_GOES_HERE
  Scope2 : Scope  NumInputPorts=9
  addr_str_0_0 : xbsIndex_r4/Constant  const=addr_str_0_0  gui_display_data_type=Fixed-point  arith_type=Unsigned  n_bits=9  bin_pt=0  preci_type=Single  exp_width=8  frac_width=24  explicit_period=on  period=1  equ=P=C  opselect=C  inp2=PCIN>>17  opr=+  inp1=P  carry=CIN  dbl_ovrd=off  block_type=constant
  addr_str_0_1 : xbsIndex_r4/Constant  const=addr_str_0_1  gui_display_data_type=Fixed-point  arith_type=Unsigned  n_bits=9  bin_pt=0  preci_type=Single  exp_width=8  frac_width=24  explicit_period=on  period=1  equ=P=C  opselect=C  inp2=PCIN>>17  opr=+  inp1=P  carry=CIN  dbl_ovrd=off  block_type=constant
  addr_str_0_2 : xbsIndex_r4/Constant  const=addr_str_0_2  gui_display_data_type=Fixed-point  arith_type=Unsigned  n_bits=9  bin_pt=0  preci_type=Single  exp_width=8  frac_width=24  explicit_period=on  period=1  equ=P=C  opselect=C  inp2=PCIN>>17  opr=+  inp1=P  carry=CIN  dbl_ovrd=off  block_type=constant
  addr_str_0_3 : xbsIndex_r4/Constant  const=addr_str_0_3  gui_display_data_type=Fixed-point  arith_type=Unsigned  n_bits=9  bin_pt=0  preci_type=Single  exp_width=8  frac_width=24  explicit_period=on  period=1  equ=P=C  opselect=C  inp2=PCIN>>17  opr=+  inp1=P  carry=CIN  dbl_ovrd=off  block_type=constant
  prg{12..22} (11 alike) : xbsIndex_r4/Delay  rst=off  infoeditControl=Selection of Reset will increase slice count due to use of real FFs and instead of SRLs  en=off  latency=1  reg_retiming=on  dbl_ovrd=off  block_type=delay
      settings: infoedit=Hardware notes: A delay line is a chain, each link of which is an SRL16 followed by a flip-flop. If register retiming is enabled, the delay line is a chain of flip-flops.  block_version=8.2-EVAL
  acc : Outport
  Out1 : Outport  Port=2
  strb : Outport  Port=3
  wires:
  addr_str_0_0/1 -> Relational1/2
  addr_str_0_1/1 -> Relational2/2
  addr_str_0_2/1 -> Relational3/2
  addr_str_0_3/1 -> Relational4/2
  count_in/1 -> Relational2/1, Relational3/1, Relational4/1, Relational1/1, Scope2/1
  Relational1/1 -> Logical1/1
  Relational2/1 -> Logical1/2
  Relational3/1 -> Logical1/3
  Relational4/1 -> Logical1/4
  prg15/1 -> Logical2/8, prg16/1
  prg12/1 -> prg15/1, Logical2/7
  Logical2/1 -> Counter1/1
  prg21/1 -> prg12/1, Logical2/6
  prg20/1 -> prg21/1, Logical2/5
  prg19/1 -> prg20/1, Logical2/4
  prg18/1 -> prg19/1, Logical2/3
  prg17/1 -> prg18/1, Logical2/2
  Logical1/1 -> Logical2/1, Counter2/1, Scope2/2, strb/1, prg17/1
  prg16/1 -> prg22/1, Logical2/9
  prg22/1 -> prg13/1, Logical2/10
  prg13/1 -> prg14/1, Logical2/11
  prg14/1 -> Logical2/12
  Counter1/1 -> Out1/1, Scope2/3
  Counter2/1 -> acc/1, Scope2/5

== system mapp_4_fir_4_str/mashinka_0/Force_str0/PARAMETERS/en1 ==
  In1 : Inport
  Delay : xbsIndex_r4/Delay  rst=off  infoeditControl=Selection of Reset will increase slice count due to use of real FFs and instead of SRLs  en=off  latency=1  reg_retiming=off  dbl_ovrd=off  block_type=delay
  Logical : xbsIndex_r4/Logical  logical_function=AND  inputs=2  en=off  latency=0  precision=Full  arith_type=Unsigned  n_bits=16  bin_pt=0  align_bp=on  dbl_ovrd=off  block_type=logical
  Logical1 : xbsIndex_r4/Logical  logical_function=XOR  inputs=2  en=off  latency=0  precision=Full  arith_type=Unsigned  n_bits=16  bin_pt=0  align_bp=on  dbl_ovrd=off  block_type=logical
  Out1 : Outport
  wires:
  In1/1 -> Logical/1, Delay/1, Logical1/2
  Logical/1 -> Out1/1
  Delay/1 -> Logical1/1
  Logical1/1 -> Logical/2

== system mapp_4_fir_4_str/mashinka_0/Force_str0/STRINGS0/Delay_tn1 ==
  Tn : Inport
  Convert53 : xbsIndex_r4/Convert  gui_display_data_type=Fixed-point  arith_type="Signed  (2's comp)"  n_bits=24  bin_pt=23  float_type=Single  exp_bits=8  fraction_bits=24  quantization=Truncate  overflow=Wrap  en=off  latency=0  pipeline=off  dbl_ovrd=off  block_type=convert
  Convert56 : xbsIndex_r4/Convert  gui_display_data_type=Floating-point  arith_type=Floating-point  n_bits=16  bin_pt=14  float_type=Single  exp_bits=8  fraction_bits=24  quantization=Truncate  overflow=Wrap  en=off  latency=8  pipeline=off  dbl_ovrd=off  block_type=convert
  curr1 : xbsIndex_r4/Delay  rst=off  infoeditControl=Selection of Reset will increase slice count due to use of real FFs and instead of SRLs  en=off  latency=24  reg_retiming=on  dbl_ovrd=off  block_type=delay
      settings: xl_area=[16 32 0 0 0 0 0]  block_version=VER_STRING_GOES_HERE
  curr67 : xbsIndex_r4/Delay  rst=off  infoeditControl=Selection of Reset will increase slice count due to use of real FFs and instead of SRLs  en=off  latency=1  reg_retiming=on  dbl_ovrd=off  block_type=delay
      settings: xl_area=[16 32 0 0 0 0 0]  block_version=VER_STRING_GOES_HERE
  curr71 : xbsIndex_r4/Delay  rst=off  infoeditControl=Selection of Reset will increase slice count due to use of real FFs and instead of SRLs  en=off  latency=1  reg_retiming=on  dbl_ovrd=off  block_type=delay
      settings: xl_area=[16 32 0 0 0 0 0]  block_version=VER_STRING_GOES_HERE
  Out1 : Outport
  wires:
  Convert56/1 -> curr71/1
  curr67/1 -> Convert56/1
  curr71/1 -> curr1/1
  Convert53/1 -> curr67/1
  Tn/1 -> Convert53/1
  curr1/1 -> Out1/1

== system mapp_4_fir_4_str/mashinka_0/Force_str0/STRINGS0/Subsystem1 ==
  In1 : Inport
  Counter : xbsIndex_r4/Counter  cnt_type=Count Limited  cnt_to=4  operation=Up  start_count=0  cnt_by_val=1  arith_type=Unsigned  n_bits=3  bin_pt=0  load_pin=off  rst=off  en=on  explicit_period=on  period=1  use_behavioral_HDL=off  implementation=Fabric  use_rpm=off  dbl_ovrd=off  block_type=counter
      settings: block_version=8.2.02
  Delay{1..3,18} (4 alike) : xbsIndex_r4/Delay  rst=off  infoeditControl=Selection of Reset will increase slice count due to use of real FFs and instead of SRLs  en=off  latency=1  reg_retiming=on  dbl_ovrd=off  block_type=delay
      settings: infoedit=Hardware notes: A delay line is a chain, each link of which is an SRL16 followed by a flip-flop. If register retiming is enabled, the delay line is a chain of flip-flops.  xl_area=[24 48 0 48 0 0 0]  block_version=VER_STRING_GOES_HERE
  Logical1 : xbsIndex_r4/Logical  logical_function=OR  inputs=5  en=off  latency=0  precision=Full  arith_type=Unsigned  n_bits=8  bin_pt=2  align_bp=on  dbl_ovrd=off  block_type=logical
      settings: xl_area=[1 0 0 1 0 0 0]  block_version=VER_STRING_GOES_HERE
  Out1 : Outport
  wires:
  Delay1/1 -> Logical1/3, Delay2/1
  Delay18/1 -> Delay1/1, Logical1/2
  Logical1/1 -> Counter/1
  In1/1 -> Delay18/1, Logical1/1
  Counter/1 -> Out1/1
  Delay2/1 -> Logical1/4, Delay3/1
  Delay3/1 -> Logical1/5
